simulink model "simulation_ex5"  (R2023a)
settings: Solver=VariableStepAuto  StartTime=0.0  StopTime=10.0  RelTol=1e-3
values from neighbouring files (symbols this model uses):
  A = [-2 1 0 0 ... (first row only)    [ex02.m]    (also in ex03.m = [-2 1 -2 0; ex04.m = [-3 3 -3; ex05.m = [zeros(2,2) eye(2); ex11.m = [-7 3 0; -6 2 -2; -2 1 -1])
  B = [0; 0; 1; 1]    [ex02.m]    (also in ex04.m = [5; -3; -2]; ex05.m = [0; 0; 1/m1; 0]; ex11.m = [3 -1; 0 0; 1 -2]; ex11_2.m = [1 0; 1 0; 0 1])
  C = [0 0 0 1]    [ex03.m]    (also in ex04.m = [1 -5 -2]; ex05.m = [1 0 0 0; 0 1 0 0]; ex11.m = [1 1 -1; 3 0 3]; ex11_2.m = [1 0 1)
  F = place(A,B,p)    [ex05.m]    (also in ex09.m = -R'*b'*P(1,1))
  L = place(A',C',[-7,-7,-6,-6])'    [ex05.m]    (also in ex06.m = place(A',C',[-6;-2;-1])'; ex06_2.m = tf([4 14 100], [1]))
settings Model: Creator=vigro  LastModifiedBy=vigro

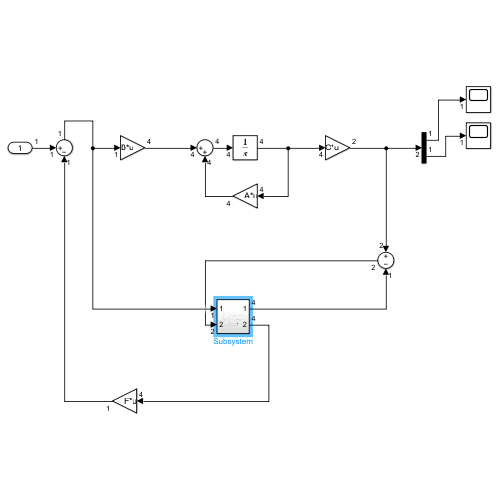
[thumbnail: Simulink's stored preview of the top-level diagram]
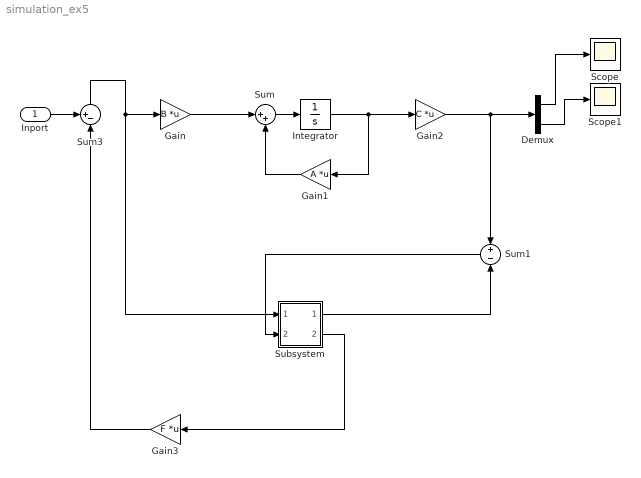
== system simulation_ex5 ==
  Inport : Inport
  Demux : Demux  Outputs=2
  Gain : Gain  Gain=B  Multiplication=Matrix(K*u)
  Gain1 : Gain  Gain=A  Multiplication=Matrix(K*u)
  Gain2 : Gain  Gain=C  Multiplication=Matrix(K*u)
  Gain3 : Gain  Gain=F  Multiplication=Matrix(K*u)
  Integrator : Integrator
  Scope : Scope
  Scope1 : Scope
  Subsystem : Subsystem
  Sum : Sum  Inputs=|++
  Sum1 : Sum  Inputs=+|-
  Sum3 : Sum  Inputs=+-|
  wires:
  Gain/1 -> Sum/1
  Sum/1 -> Integrator/1
  Integrator/1 -> Gain1/1, Gain2/1
  Gain1/1 -> Sum/2
  Gain2/1 -> Demux/1, Sum1/1
  Sum3/1 -> Subsystem/1(In1), Gain/1
  Inport/1 -> Sum3/1
  Gain3/1 -> Sum3/2
  Demux/1 -> Scope/1
  Demux/2 -> Scope1/1
  Subsystem/1(Out1) -> Sum1/2
  Sum1/1 -> Subsystem/2(In2)
  Subsystem/2(Out2) -> Gain3/1

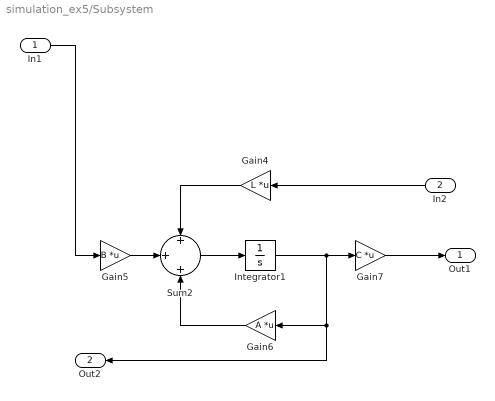
== system simulation_ex5/Subsystem ==
  In1 : Inport
  In2 : Inport  Port=2
  Gain4 : Gain  Gain=L  Multiplication=Matrix(K*u)
  Gain5 : Gain  Gain=B  Multiplication=Matrix(K*u)
  Gain6 : Gain  Gain=A  Multiplication=Matrix(K*u)
  Gain7 : Gain  Gain=C  Multiplication=Matrix(K*u)
  Integrator1 : Integrator
  Sum2 : Sum  Inputs=+|+|+
  Out1 : Outport
  Out2 : Outport  Port=2
  wires:
  Integrator1/1 -> Out2/1, Gain6/1, Gain7/1
  Gain4/1 -> Sum2/1
  In2/1 -> Gain4/1
  In1/1 -> Gain5/1
  Gain6/1 -> Sum2/3
  Gain7/1 -> Out1/1
  Gain5/1 -> Sum2/2
  Sum2/1 -> Integrator1/1
